simulink subsystem "flag_GC"  (R2024a)
settings: Solver=VariableStepAuto  StartTime=0.0  StopTime=10.0  RelTol=1e-3
libraries: px4lib x1
settings Model: Creator=gurt1  LastModifiedBy=gurt1

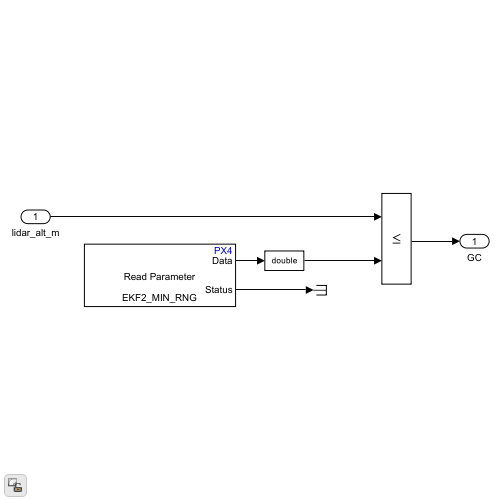
[thumbnail: Simulink's stored preview of the top-level diagram]
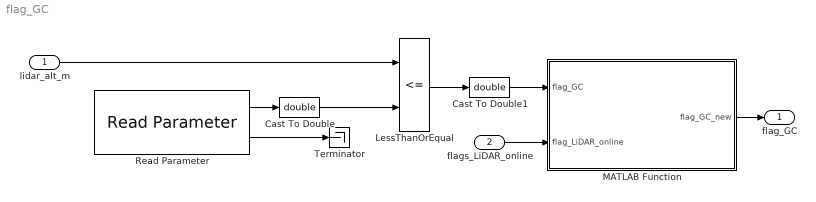
== system flag_GC ==
  lidar_alt_m : Inport
  flags_LiDAR_online : Inport  Port=2
  Cast To Double : DataTypeConversion  OutDataTypeStr=double  SaturateOnIntegerOverflow=off  RndMeth=Floor
  Cast To Double1 : DataTypeConversion  OutDataTypeStr=double  SaturateOnIntegerOverflow=off  RndMeth=Floor
  LessThanOrEqual : RelationalOperator  Operator=<=  RndMeth=Simplest  InputSameDT=off
  MATLAB Function : MATLAB Function  TreatAsAtomicUnit=on
  Read Parameter : px4lib/Read Parameter  ParameterName=EKF2_MIN_RNG  DataType=FLOAT  SampleTime=-1
  Terminator : Terminator
  flag_GC : Outport
  wires:
  Read Parameter/2 -> Terminator/1
  Read Parameter/1 -> Cast To Double/1
  lidar_alt_m/1 -> LessThanOrEqual/1
  Cast To Double/1 -> LessThanOrEqual/2
  LessThanOrEqual/1 -> Cast To Double1/1
  Cast To Double1/1 -> MATLAB Function/1(flag_GC)
  MATLAB Function/1(flag_GC_new) -> flag_GC/1
  flags_LiDAR_online/1 -> MATLAB Function/2(flag_LiDAR_online)

== matlab function flag_GC/MATLAB Function ==
  data: flag_GC input; flag_LiDAR_online input; flag_GC_new output
function flag_GC_new = LiDAR_status_check(flag_GC,flag_LiDAR_online)
% This logic checks to see if the LiDAR module is available before
% determining if the vehicle has landed or not.

if flag_LiDAR_online >= 0.5
    flag_GC_new = flag_GC;
else 
    flag_GC_new = 0;
end
